simulink model "WAMV_Control"  (R2024a)
settings: Solver=FixedStepAuto  StartTime=0.0  StopTime=Inf  RelTol=1e-3
undefined symbols (not defined in the file): goalPos, waypoints
libraries: ros2lib x6, robotalgslib x1, sharedtransform x1
settings Model: Creator=abshanka  LastModifiedBy=abshanka
settings OptimizationCC: EnhancedBackFolding=on  PassReuseOutputArgsAs=Individual arguments  ZeroExternalMemoryAtStartup=off  ZeroInternalMemoryAtStartup=off  MaxStackSize=64  OptimizeBlockOrder=speed  DifferentSizesBufferReuse=on  OptimizationCustomize=off  EfficientTunableParamExpr=on
settings DebuggingCC: ParameterTunabilityLossMsg=error
settings SFSimCC: MATLABDynamicMemAlloc=off
settings RTWCC: Description=Embedded Coder  SystemTargetFile=ert.tlc  HardwareBoard=Robot Operating System 2 (ROS 2)  TLCOptions="-aInlineSetEventsForThisBaseRateFcn=TLC_FALSE -aSuppressMultiTaskScheduler=TLC_FALSE  -aRateBasedStepFcn=0"  GenCodeOnly=on  TemplateMakefile=ert_default_tmf  Toolchain=Colcon Tools  TargetLang=C++
settings CodeAppCC: ForceParamTrailComments=on  IgnoreCustomStorageClasses=off  OperatorAnnotations=on  SimulinkDataObjDesc=on  SFDataObjDesc=on  InsertBlockDesc=on
settings ERTTargetCC: CodeInterfacePackaging=C++ class  RootIOFormat=Structure reference

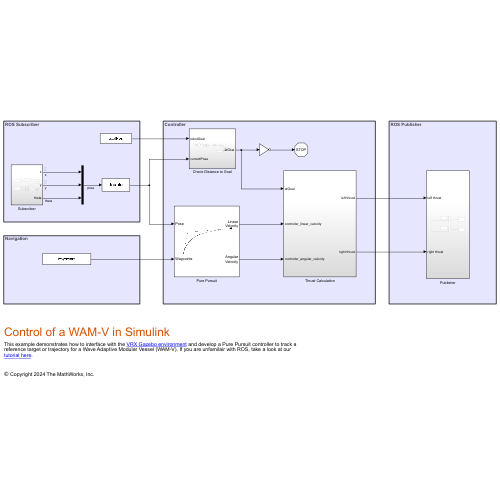
[thumbnail: Simulink's stored preview of the top-level diagram]
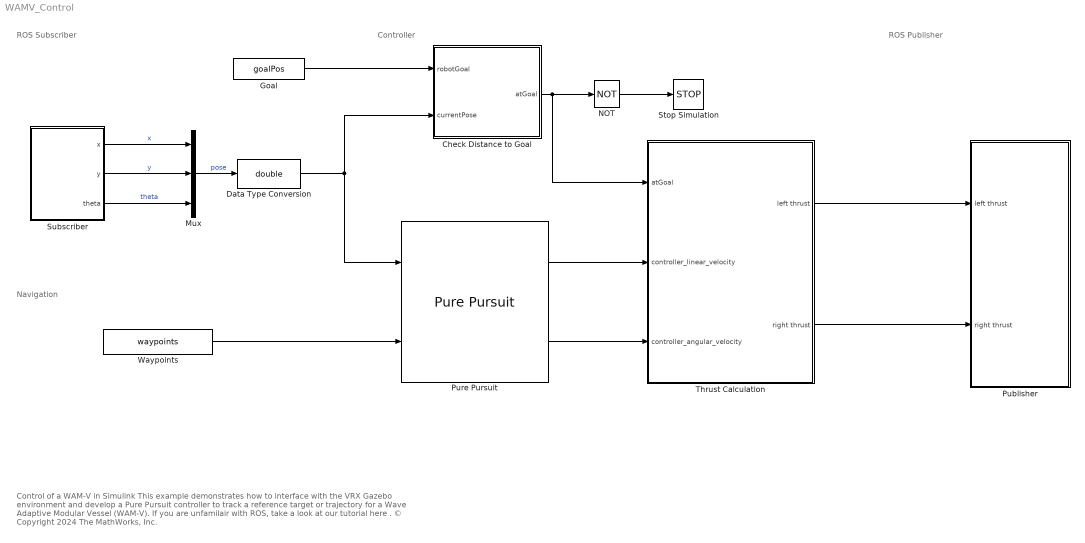
== system WAMV_Control ==
  note: Navigation
  note: ROS Publisher
  note: ROS Subscriber
  note: Controller
  note: Control of a WAM-V in Simulink
      | This example demonstrates how to interface with the VRX Gazebo environment and develop a Pure Pursuit controller to track a reference target or trajectory for a Wave Adaptive Modular Vessel (WAM-V). If you are unfamilair with ROS, take a look at our tutorial here .
      |
      | © Copyright 2024 The MathWorks, Inc.
  Check Distance to Goal : Subsystem
  Data Type Conversion : DataTypeConversion  OutDataTypeStr=double  SaturateOnIntegerOverflow=off  RndMeth=Floor
  Goal : Constant  Value=goalPos
  Mux : Mux  Inputs=3
  NOT : Logic  Operator=NOT  IconShape=distinctive  AllPortsSameDT=off  OutDataTypeStr=boolean
  Publisher : Subsystem
  Pure Pursuit : robotalgslib/Pure Pursuit  DesiredLinearVelocityPort=off  DesiredLinearVelocity=0.3  MaxAngularVelocity=0.4  LookaheadDistancePort=off  LookaheadDistance=5  TargetDirPort=off  SimulateUsing=Code generation
      settings: LibrarySourceBlock=navlib/Control Algorithms/Pure Pursuit
  Stop Simulation : Stop
  Subscriber : Subsystem
  Thrust Calculation : Subsystem
  Waypoints : Constant  Value=waypoints
  wires:
  Subscriber/1(x) -> Mux/1  "x"
  Subscriber/2(y) -> Mux/2  "y"
  Subscriber/3(theta) -> Mux/3  "theta"
  Mux/1 -> Data Type Conversion/1  "pose"
  Data Type Conversion/1 -> Check Distance to Goal/2(currentPose), Pure Pursuit/1
  Check Distance to Goal/1(atGoal) -> Thrust Calculation/1(atGoal), NOT/1
  NOT/1 -> Stop Simulation/1
  Thrust Calculation/1(left thrust) -> Publisher/1(left thrust)
  Thrust Calculation/2(right thrust) -> Publisher/2(right thrust)
  Waypoints/1 -> Pure Pursuit/2
  Goal/1 -> Check Distance to Goal/1(robotGoal)
  Pure Pursuit/1 -> Thrust Calculation/2(controller_linear_velocity)
  Pure Pursuit/2 -> Thrust Calculation/3(controller_angular_velocity)

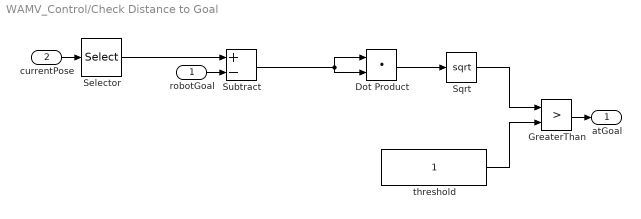
== system WAMV_Control/Check Distance to Goal ==
  robotGoal : Inport
  currentPose : Inport  Port=2
  Dot Product : DotProduct  OutDataTypeStr=Inherit: Inherit via internal rule
  GreaterThan : RelationalOperator  Operator=>  OutDataTypeStr=boolean  RndMeth=Simplest  InputSameDT=off
  Selector : Selector  InputPortWidth=3  IndexOptions=Index vector (dialog)  Indices=[1 2]  OutputSizes=1
  Sqrt : Sqrt
  Subtract : Sum  Inputs=+-
  threshold : Constant
  atGoal : Outport
  wires:
  currentPose/1 -> Selector/1
  robotGoal/1 -> Subtract/2
  Selector/1 -> Subtract/1
  Subtract/1 -> Dot Product/2, Dot Product/1
  Sqrt/1 -> GreaterThan/1
  GreaterThan/1 -> atGoal/1
  threshold/1 -> GreaterThan/2
  Dot Product/1 -> Sqrt/1

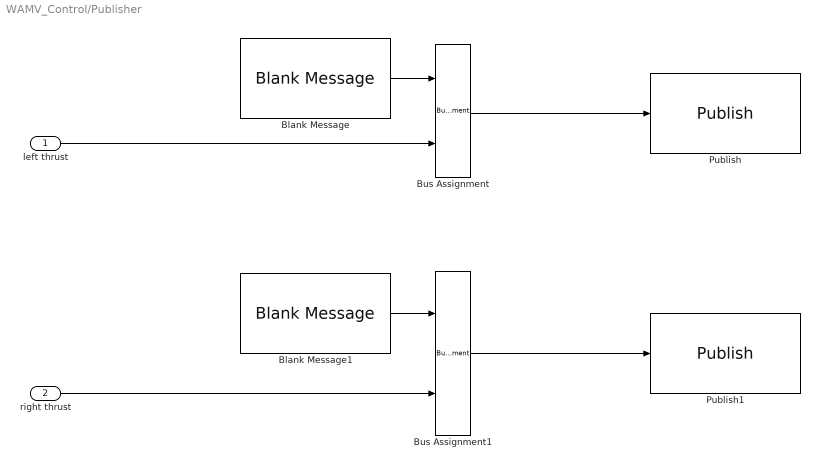
== system WAMV_Control/Publisher ==
  left thrust : Inport
  right thrust : Inport  Port=2
  Blank Message : ros2lib/Blank Message  messageClass=Message  entityType=std_msgs/Float64  messageType=std_msgs/Float64  SampleTime=inf
  Blank Message1 : ros2lib/Blank Message  messageClass=Message  entityType=std_msgs/Float64  messageType=std_msgs/Float64  SampleTime=inf
  Bus Assignment : BusAssignment  AssignedSignals=data
  Bus Assignment1 : BusAssignment  AssignedSignals=data
  Publish : ros2lib/Publish  topicSource=Select from ROS network  topic=/wamv/thrusters/left/thrust  messageType=std_msgs/Float64  QOSHistory=Keep last  QOSDepth=1  QOSReliability=Reliable  QOSDurability=Volatile  QOSDeadline=Inf  QOSLifespan=Inf  QOSLiveliness=Automatic  QOSLeaseDuration=Inf  QOSAvoidROSNamespaceConventions=off
  Publish1 : ros2lib/Publish  topicSource=Select from ROS network  topic=/wamv/thrusters/right/thrust  messageType=std_msgs/Float64  QOSHistory=Keep last  QOSDepth=1  QOSReliability=Reliable  QOSDurability=Volatile  QOSDeadline=Inf  QOSLifespan=Inf  QOSLiveliness=Automatic  QOSLeaseDuration=Inf  QOSAvoidROSNamespaceConventions=off
  wires:
  Blank Message/1 -> Bus Assignment/1
  right thrust/1 -> Bus Assignment1/2
  Bus Assignment/1 -> Publish/1
  Bus Assignment1/1 -> Publish1/1
  left thrust/1 -> Bus Assignment/2
  Blank Message1/1 -> Bus Assignment1/1

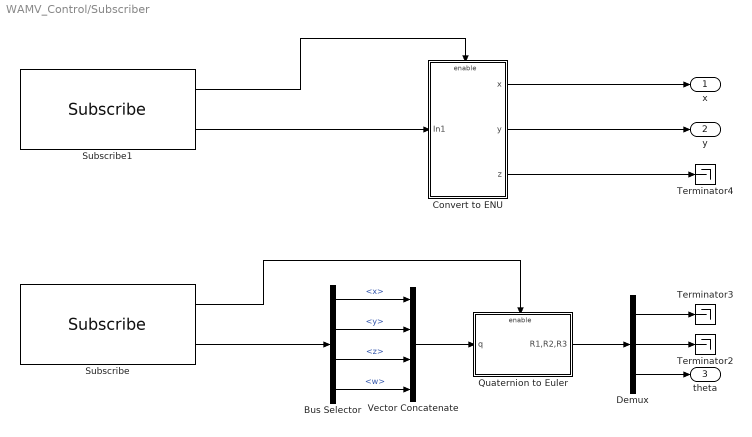
== system WAMV_Control/Subscriber ==
  Bus Selector : BusSelector  OutputSignals=orientation.x,orientation.y,orientation.z,orientation.w
  Convert to ENU : Subsystem
  Demux : Demux  Outputs=3
  Quaternion to Euler : Subsystem
  Subscribe : ros2lib/Subscribe  topicSource=Select from ROS network  topic=/wamv/sensors/imu/imu/data  messageType=sensor_msgs/Imu  sampleTime=-1  QOSHistory=Keep last  QOSDepth=1  QOSReliability=Reliable  QOSDurability=Volatile  QOSDeadline=Inf  QOSLifespan=Inf  QOSLiveliness=Automatic  QOSLeaseDuration=Inf  QOSAvoidROSNamespaceConventions=off
  Subscribe1 : ros2lib/Subscribe  topicSource=Select from ROS network  topic=/wamv/sensors/gps/gps/fix  messageType=sensor_msgs/NavSatFix  sampleTime=-1  QOSHistory=Keep last  QOSDepth=1  QOSReliability=Reliable  QOSDurability=Volatile  QOSDeadline=Inf  QOSLifespan=Inf  QOSLiveliness=Automatic  QOSLeaseDuration=Inf  QOSAvoidROSNamespaceConventions=off
  Terminator2 : Terminator
  Terminator3 : Terminator
  Terminator4 : Terminator
  Vector Concatenate : Concatenate  NumInputs=4
  x : Outport
  y : Outport  Port=2
  theta : Outport  Port=3
  wires:
  Subscribe/2 -> Bus Selector/1
  Subscribe/1 -> Quaternion to Euler/Enable
  Subscribe1/1 -> Convert to ENU/Enable
  Bus Selector/1 -> Vector Concatenate/1  "<x>"
  Bus Selector/2 -> Vector Concatenate/2  "<y>"
  Bus Selector/3 -> Vector Concatenate/3  "<z>"
  Bus Selector/4 -> Vector Concatenate/4  "<w>"
  Demux/1 -> Terminator3/1
  Demux/2 -> Terminator2/1
  Demux/3 -> theta/1
  Vector Concatenate/1 -> Quaternion to Euler/1(q)
  Quaternion to Euler/1(R1,R2,R3) -> Demux/1
  Subscribe1/2 -> Convert to ENU/1(In1)
  Convert to ENU/1(x) -> x/1
  Convert to ENU/2(y) -> y/1
  Convert to ENU/3(z) -> Terminator4/1

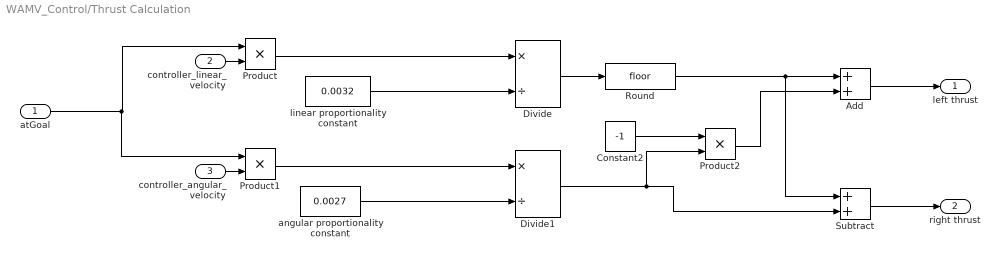
== system WAMV_Control/Thrust Calculation ==
  atGoal : Inport
  controller_linear_velocity : Inport  Port=2
  controller_angular_velocity : Inport  Port=3
  Add : Sum
  Constant2 : Constant  Value=-1
  Divide : Product  Inputs=*/
  Divide1 : Product  Inputs=*/
  Product : Product
  Product1 : Product
  Product2 : Product
  Round : Rounding
  Subtract : Sum
  angular proportionality constant : Constant  Value=0.0027
  linear proportionality constant : Constant  Value=0.0032
  left thrust : Outport
  right thrust : Outport  Port=2
  wires:
  atGoal/1 -> Product1/1, Product/1
  Product/1 -> Divide/1
  controller_angular_velocity/1 -> Product1/2
  controller_linear_velocity/1 -> Product/2
  Round/1 -> Subtract/1, Add/1
  linear proportionality constant/1 -> Divide/2
  Product1/1 -> Divide1/1
  Divide/1 -> Round/1
  Add/1 -> left thrust/1
  Subtract/1 -> right thrust/1
  angular proportionality constant/1 -> Divide1/2
  Divide1/1 -> Product2/2, Subtract/2
  Product2/1 -> Add/2
  Constant2/1 -> Product2/1

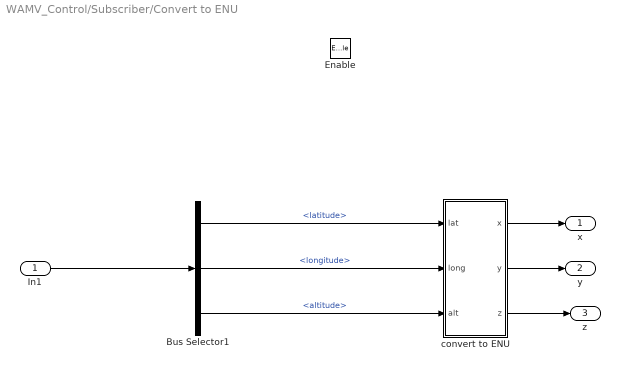
== system WAMV_Control/Subscriber/Convert to ENU ==
  In1 : Inport
  Enable : EnablePort
  Bus Selector1 : BusSelector  OutputSignals=latitude,longitude,altitude
  convert to ENU : MATLAB Function  TreatAsAtomicUnit=on
  x : Outport
  y : Outport  Port=2
  z : Outport  Port=3
  wires:
  convert to ENU/3(z) -> z/1
  Bus Selector1/2 -> convert to ENU/2(long)  "<longitude>"
  convert to ENU/1(x) -> x/1
  Bus Selector1/3 -> convert to ENU/3(alt)  "<altitude>"
  Bus Selector1/1 -> convert to ENU/1(lat)  "<latitude>"
  In1/1 -> Bus Selector1/1
  convert to ENU/2(y) -> y/1

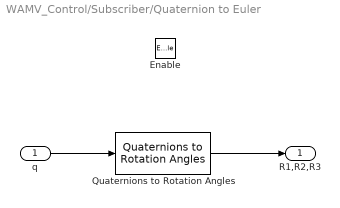
== system WAMV_Control/Subscriber/Quaternion to Euler ==
  q : Inport
  Enable : EnablePort
  Quaternions to Rotation Angles : sharedtransform/Quaternions to Rotation Angles  rotationOrder=ZYX  aMode=aMode
  R1,R2,R3 : Outport
  wires:
  q/1 -> Quaternions to Rotation Angles/1
  Quaternions to Rotation Angles/1 -> R1,R2,R3/1

== matlab function WAMV_Control/Subscriber/Convert to ENU/convert to ENU ==
  data: x output; lat input; y output; long input; alt input; z output
function [x, y, z] = gps2enu(lat, long, alt)

wgs84 = wgs84Ellipsoid;
lat0 = -33.724223;
long0 = 150.679736;
alt0 = 0;

[x, y, z] = geodetic2enu(lat, long, alt, lat0, long0, alt0, wgs84);
